simulink model "taller1_entregable"  (R2020a)
settings: Solver=VariableStepAuto  StartTime=0.0  StopTime=5  RelTol=1e-3
values from neighbouring files (symbols this model uses):
  K = media/max(in)    [taller_1.m]
  tau = xhigh-xlow    [taller_1.m]
  tauan = 1.5*(x63-x28)    [taller_1.m]
  taumiller = data.time(data.system_response>= ymiller-0.01 & data.system_response<= ymiller+0.01)-theta    [taller_1.m]
  theta = xlow    [taller_1.m]
  thetan = x63-tauan    [taller_1.m]
settings Model: Creator=Personal  LastModifiedBy=Personal

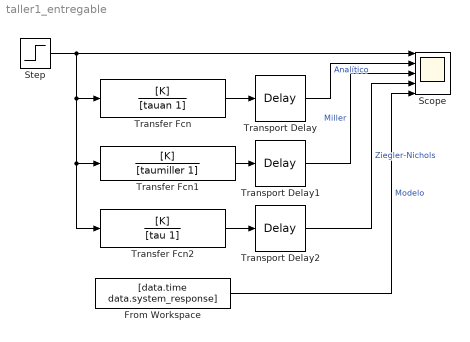
== system taller1_entregable ==
  From Workspace : FromWorkspace  VariableName=[data.time data.system_response]
  Scope : Scope  NumInputPorts=5
  Step : Step  Time=0.2021  After=1.5  SampleTime=0
  Transfer Fcn : TransferFcn  Numerator=[K]  Denominator=[tauan 1]
  Transfer Fcn1 : TransferFcn  Numerator=[K]  Denominator=[taumiller 1]
  Transfer Fcn2 : TransferFcn  Numerator=[K]  Denominator=[tau 1]
  Transport Delay : TransportDelay  DelayTime=thetan
  Transport Delay1 : TransportDelay  DelayTime=theta
  Transport Delay2 : TransportDelay  DelayTime=theta
  wires:
  Transfer Fcn/1 -> Transport Delay/1
  Transport Delay/1 -> Scope/2  "Analítico"
  From Workspace/1 -> Scope/5  "Modelo"
  Transfer Fcn1/1 -> Transport Delay1/1
  Transfer Fcn2/1 -> Transport Delay2/1
  Step/1 -> Transfer Fcn2/1, Transfer Fcn1/1, Transfer Fcn/1, Scope/1
  Transport Delay1/1 -> Scope/3  "Miller"
  Transport Delay2/1 -> Scope/4  "Ziegler-Nichols"
